simulink model "prop_tilt_gyro_model_1"  (R2020b)
settings: Solver=VariableStepAuto  StartTime=0.0  StopTime=10.0  RelTol=1e-3
values from neighbouring files (symbols this model uses):
  I_mat = [2 10 0 ... (first row only)    [Propellers_tilt.m]    (also in tilt_verification.m = 0)
  psI_0 = 0    [tilt_verification.m]
  psI_dot = 0    [tilt_verification.m]
  w_p_0 = 90*pi/(180*T_prop)    (= 1.57079632679)    [tilt_verification.m]
  w_p_dot = 0    [tilt_verification.m]
  w_s_0 = 3500*2*pi/2    (= 10995.5742876)    [tilt_verification.m]
  w_s_dot = 0    [tilt_verification.m]
libraries: sharedutil x1
settings Model: Creator=Jonathan van Zyl  LastModifiedBy=Jonathan van Zyl

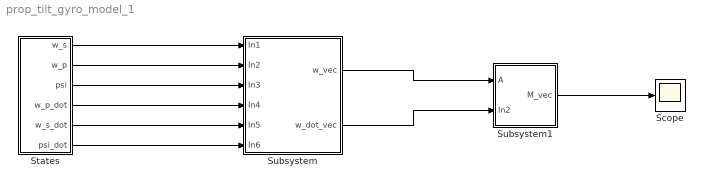
== system prop_tilt_gyro_model_1 ==
  Scope : Scope
  States : Subsystem
  Subsystem : Subsystem
  Subsystem1 : Subsystem
  wires:
  States/1(w_s) -> Subsystem/1(In1)
  States/2(w_p) -> Subsystem/2(In2)
  States/3(psi) -> Subsystem/3(In3)
  States/4(w_p_dot) -> Subsystem/4(In4)
  States/5(w_s_dot) -> Subsystem/5(In5)
  States/6(psi_dot) -> Subsystem/6(In6)
  Subsystem/1(w_vec) -> Subsystem1/1(A)
  Subsystem/2(w_dot_vec) -> Subsystem1/2(In2)
  Subsystem1/1(M_vec) -> Scope/1

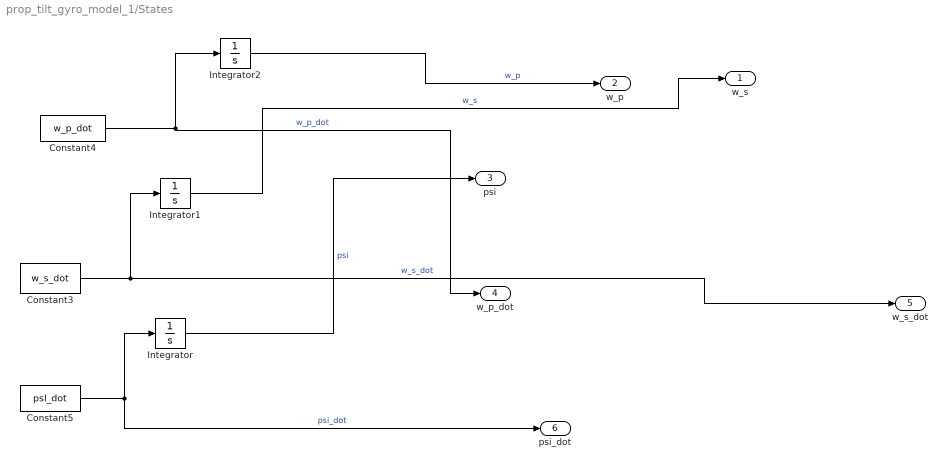
== system prop_tilt_gyro_model_1/States ==
  Constant3 : Constant  Value=w_s_dot
  Constant4 : Constant  Value=w_p_dot
  Constant5 : Constant  Value=psI_dot
  Integrator : Integrator  InitialCondition=psI_0
  Integrator1 : Integrator  InitialCondition=w_s_0
  Integrator2 : Integrator  InitialCondition=w_p_0
  w_s : Outport
  w_p : Outport  Port=2
  psi : Outport  Port=3
  w_p_dot : Outport  Port=4
  w_s_dot : Outport  Port=5
  psi_dot : Outport  Port=6
  wires:
  Integrator2/1 -> w_p/1  "w_p"
  Integrator1/1 -> w_s/1  "w_s"
  Constant5/1 -> psi_dot/1, Integrator/1  "psi_dot"
  Integrator/1 -> psi/1  "psi"
  Constant4/1 -> w_p_dot/1, Integrator2/1  "w_p_dot"
  Constant3/1 -> w_s_dot/1, Integrator1/1  "w_s_dot"

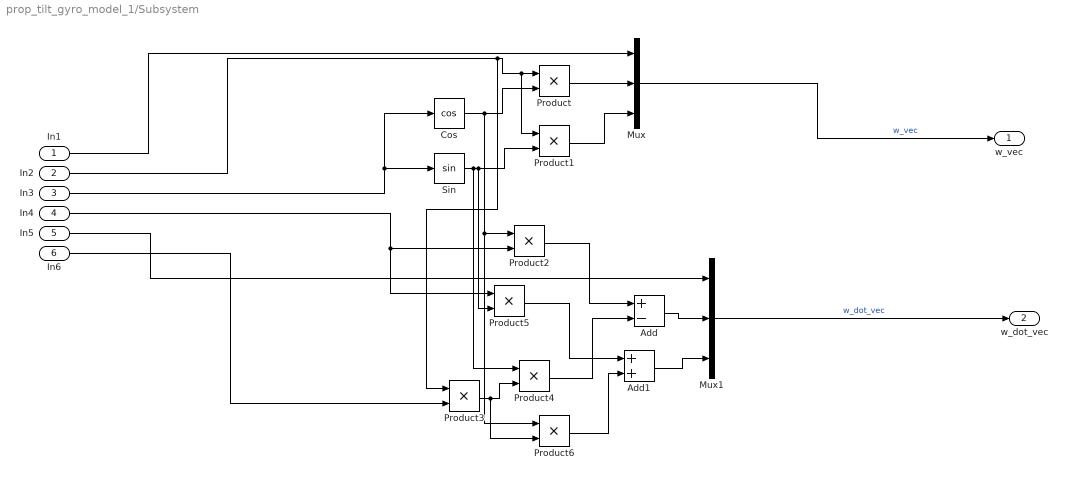
== system prop_tilt_gyro_model_1/Subsystem ==
  In1 : Inport
  In2 : Inport  Port=2
  In3 : Inport  Port=3
  In4 : Inport  Port=4
  In5 : Inport  Port=5
  In6 : Inport  Port=6
  Add : Sum  Inputs=+-
  Add1 : Sum
  Cos : Trigonometry  Operator=cos
  Mux : Mux  Inputs=3
  Mux1 : Mux  Inputs=3
  Product{,1..6} (7 alike) : Product
  Sin : Trigonometry
  w_vec : Outport
  w_dot_vec : Outport  Port=2
  wires:
  Add/1 -> Mux1/2
  Product3/1 -> Product6/2, Product4/2
  In2/1 -> Product3/1, Product1/1, Product/1
  Product2/1 -> Add/1
  Cos/1 -> Product6/1, Product2/1, Product/2
  In3/1 -> Cos/1, Sin/1
  Sin/1 -> Product4/1, Product5/2, Product1/2
  In4/1 -> Product5/1, Product2/2
  Product6/1 -> Add1/2
  Add1/1 -> Mux1/3
  Product/1 -> Mux/2
  Mux/1 -> w_vec/1  "w_vec"
  Product5/1 -> Add1/1
  Product4/1 -> Add/2
  Product1/1 -> Mux/3
  In1/1 -> Mux/1
  In6/1 -> Product3/2
  Mux1/1 -> w_dot_vec/1  "w_dot_vec"
  In5/1 -> Mux1/1

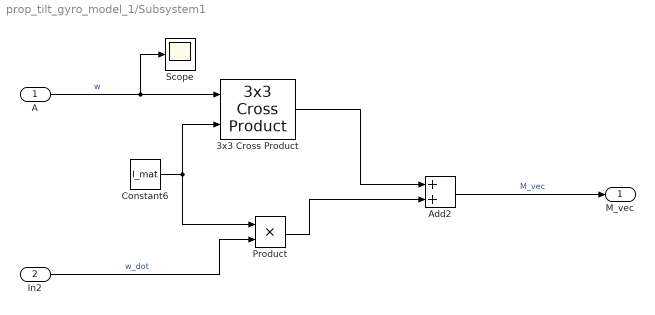
== system prop_tilt_gyro_model_1/Subsystem1 ==
  A : Inport
  In2 : Inport  Port=2
  3x3 Cross Product : sharedutil/3x3 Cross Product  aMode=aMode
      settings: SourceProductBaseCode=AE,PW,MT,UV,VE,VP
  Add2 : Sum
  Constant6 : Constant  Value=I_mat
  Product : Product
  Scope : Scope
  M_vec : Outport
  wires:
  Product/1 -> Add2/2
  In2/1 -> Product/2  "w_dot"
  A/1 -> Scope/1, 3x3 Cross Product/1  "w"
  Constant6/1 -> Product/1, 3x3 Cross Product/2
  3x3 Cross Product/1 -> Add2/1
  Add2/1 -> M_vec/1  "M_vec"
